simulink model "ammclib_gflib_limit_s32k11x"  (Simulink 9.0)
settings: Solver=FixedStepDiscrete  StartTime=0.0  StopTime=5  FixedStep=0.1  RelTol=1e-3  EnableMultiTasking=on
InitFcn:
  | mbd_s32k_consistency_checks(bdroot(gcs));
undefined symbols (not defined in the file): LQFP, thumb
libraries: simulink x11, ammclib_bam_s32k11x x10, mbd_s32k1xx_ec_toolbox x2
Description:
  | This model tests the AMMCLIB GFLIB LIMIT blocks
  | 
  | Validation:
  | - Run the model in Simulation and check the results
  | - Open Freemaster (ammclib_gflib_limit_s32k11x.pmp) and compare the HW results against the Simulated ones
CloseFcn:
  | clear all;
settings Model: Creator=NXP MBDT Team  LastModifiedBy=nxf35172
settings DataIOCC: ExternalInput=off  InitialState=off  LimitDataPoints=on  SaveOutput=off  SignalLogging=off  SaveTime=off
settings OptimizationCC: DefaultParameterBehavior=Inlined  PassReuseOutputArgsAs=Individual arguments  LifeSpan=auto
settings DebuggingCC: SolverPrmCheckMsg=warning  InheritedTsInSrcMsg=none  SingleTaskRateTransMsg=error  IntegerOverflowMsg=none  ParameterPrecisionLossMsg=none  ParameterTunabilityLossMsg=error  UnconnectedInputMsg=error  UnconnectedOutputMsg=error  UnconnectedLineMsg=error  AllowSymbolicDim=off  UnknownTsInhSupMsg=error  StateNameClashWarn=warning
settings HardwareCC: ProdLargestAtomicInteger=Long  ProdLargestAtomicFloat=Double  ProdIntDivRoundTo=Zero  ProdEndianess=LittleEndian  ProdHWDeviceType=ARM Compatible->ARM Cortex
settings SFSimCC: MATLABDynamicMemAlloc=off
settings RTWCC: SystemTargetFile=mbd_s32k.tlc  MakeCommand=mbd_s32k_make_rtw COPY_MDLREF_INCLUDES=0  TemplateMakefile=mbd_s32k.tmf  Description=Model Based Design Toolbox S32K14x Code Generation Target  GenerateReport=on  IncludeHyperlinkInReport=on  LaunchReport=on  GenerateTraceInfo=on  GenerateTraceReport=on  GenerateTraceReportSl=on  GenerateTraceReportSf=on  GenerateTraceReportEml=on
settings CodeAppCC: ForceParamTrailComments=on  IgnoreCustomStorageClasses=off  OperatorAnnotations=on  SimulinkDataObjDesc=on  SFDataObjDesc=on  InsertBlockDesc=on  StateflowObjectComments=off
settings STFCustomTargetCC: MultiwordLength=256  ModelReferenceCompliant=off  CombineOutputUpdateFcns=on  ERTCustomFileBanners=on  SupportContinuousTime=off  SupportNonInlinedSFcns=off  RemoveResetFunc=on  MATLABClassNameForMDSCustomization=Simulink.SoftwareTarget.ERTCustomization  GRTInterface=off  SystemTargetFile=mbd_s32k.tlc
settings ERTTargetCC: ModelReferenceCompliant=off  ParMdlRefBuildCompliant=off  CompOptLevelCompliant=off  ConcurrentExecutionCompliant=off  ModelStepFunctionPrototypeControlCompliant=off  CPPClassGenCompliant=off  UseToolchainInfoCompliant=off  InlinedParameterPlacement=NonHierarchical  ERTCustomFileTemplate=example_file_process.tlc

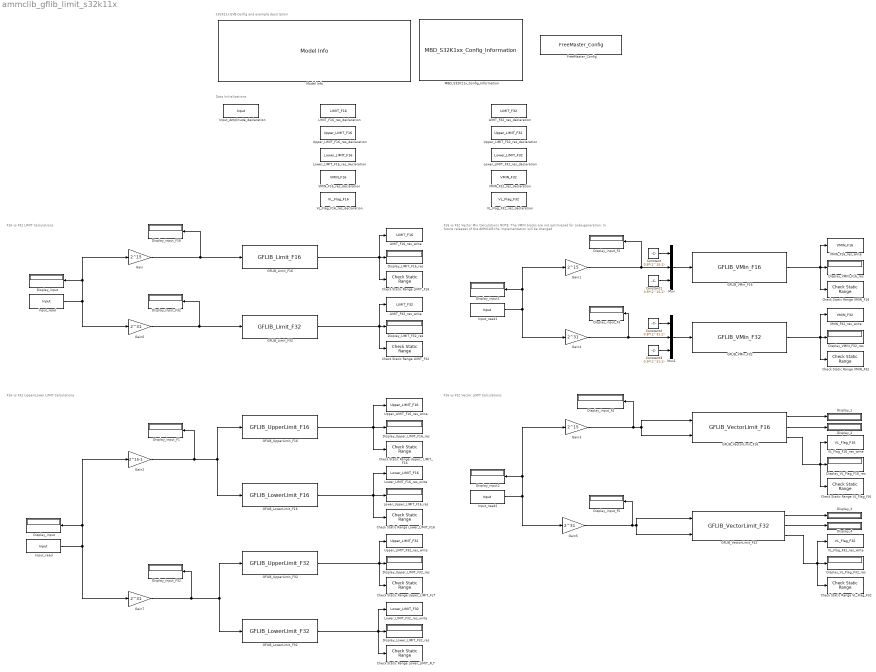
== system ammclib_gflib_limit_s32k11x ==
  note: S32K11x EVB Config and example description
  note: Data Initializations
  note: F16 vs F32 LIMIT Calculations
  note: F16 vs F32 Upper/Lower LIMIT Calculations
  note: F16 vs F32 Vector Min Calculations
      | NOTE: The VMIN blocks are not optimiezed for code-generation. In future releases of the AMMCLIB the implementation will be changed
  note: F16 vs F32 Vector LIMIT Calculations
  "Check Static Range LIMIT_F16 " : simulink/Model Verification/Check  Static Range  Description=-0.5*(2^15-1)-1 <= u <= 0.5*(2^15-1)+1  max=0.5*(2^15-1)+1  max_included=on  min=-0.5*(2^15-1)-1  min_included=on  enabled=on  stopWhenAssertionFail=on  export=off  icon=graphic
      settings: SourceProductName=Simulink  SourceProductBaseCode=SL
  Check Static Range LIMIT_F32 : simulink/Model Verification/Check  Static Range  Description=-0.5*(2^31-1)-1 <= u <= 0.5*(2^31-1)+1  max=0.5*(2^31-1)+1  max_included=on  min=-0.5*(2^31-1)-1  min_included=on  enabled=on  stopWhenAssertionFail=on  export=off  icon=graphic
      settings: SourceProductName=Simulink  SourceProductBaseCode=SL
  Check Static Range Lower_LIMIT_F16 : simulink/Model Verification/Check  Static Range  Description=-0.5*(2^15-1)-1 <= u <= (2^15-1)  max=(2^15-1)  max_included=on  min=-0.5*(2^15-1)-1  min_included=on  enabled=on  stopWhenAssertionFail=on  export=off  icon=graphic
      settings: SourceProductName=Simulink  SourceProductBaseCode=SL
  Check Static Range Lower_LIMIT_FLT : simulink/Model Verification/Check  Static Range  Description=-0.5*(2^31-1)-1 <= u <= (2^31-1)  max=(2^31-1)  max_included=on  min=-0.5*(2^31-1)-1  min_included=on  enabled=on  stopWhenAssertionFail=on  export=off  icon=graphic
      settings: SourceProductName=Simulink  SourceProductBaseCode=SL
  "Check Static Range Upper_ LIMIT_F16 " : simulink/Model Verification/Check  Static Range  Description=-(2^15-1) <= u <= 0.5*(2^15-1)+1  max=0.5*(2^15-1)+1  max_included=on  min=-(2^15-1)  min_included=on  enabled=on  stopWhenAssertionFail=on  export=off  icon=graphic
      settings: SourceProductName=Simulink  SourceProductBaseCode=SL
  Check Static Range Upper_LIMIT_FLT : simulink/Model Verification/Check  Static Range  Description=-(2^31-1) <= u <= 0.5*(2^31-1)+1  max=0.5*(2^31-1)+1  max_included=on  min=-(2^31-1)  min_included=on  enabled=on  stopWhenAssertionFail=on  export=off  icon=graphic
      settings: SourceProductName=Simulink  SourceProductBaseCode=SL
  Check Static Range VL_Flag_F32 : simulink/Model Verification/Check  Static Range  Description=0 <= u <= 1  max=1  max_included=on  min=0  min_included=on  enabled=on  stopWhenAssertionFail=on  export=off  icon=graphic
      settings: SourceProductName=Simulink  SourceProductBaseCode=SL
  Check Static Range VL_Flag_f16 : simulink/Model Verification/Check  Static Range  Description=0 <= u <= 1  max=1  max_included=on  min=0  min_included=on  enabled=on  stopWhenAssertionFail=on  export=off  icon=graphic
      settings: SourceProductName=Simulink  SourceProductBaseCode=SL
  Check Static Range VMIN_F16 : simulink/Model Verification/Check  Static Range  Description=0 <= u <= 2  max=2  max_included=on  min=0  min_included=on  enabled=on  stopWhenAssertionFail=on  export=off  icon=graphic
      settings: SourceProductName=Simulink  SourceProductBaseCode=SL
  Check Static Range VMIN_F32 : simulink/Model Verification/Check  Static Range  Description=0 <= u <= 2  max=2  max_included=on  min=0  min_included=on  enabled=on  stopWhenAssertionFail=on  export=off  icon=graphic
      settings: SourceProductName=Simulink  SourceProductBaseCode=SL
  Constant : Constant  Value=0.8*(2^15-1)  OutDataTypeStr=int16
  Constant1 : Constant  Value=0.9*(2^15-1)  OutDataTypeStr=int16
  Constant2 : Constant  Value=0.8*(2^31-1)  OutDataTypeStr=int32
  Constant3 : Constant  Value=0.9*(2^31-1)  OutDataTypeStr=int32
  Display_{1..4} (4 alike) : Display
  Display_LIMIT_F16_res : Display
  Display_LIMIT_F32_res : Display
  Display_Lower_LIMIT_F32_res : Display
  Display_Upper_LIMIT_F16_res : Display
  Display_Upper_LIMIT_F32_res : Display
  Display_VL_Flag_F16_res : Display
  Display_VL_Flag_F32_res : Display
  Display_VMIN_F16_res : Display
  Display_VMIN_F32_res : Display
  Display_input : Display
  "Display_input  " : Display
  Display_input1 : Display
  Display_input2 : Display
  Display_input_F{1..5,16,32} (7 alike) : Display
  "Display_input_F32  " : Display
  FreeMaster_Config : mbd_s32k1xx_ec_toolbox/Utility Blocks/FreeMaster_Config  interface=LPUART0  baudrate=19200  rxd=PTB0: [LPUART0_RX | Receive]  txd=PTB1: [LPUART0_TX | Transmit]  mode=Short Interrupt  isr_prio=1  show_adv_opts=on  use_scope=on  max_scope_vars=8  use_recorder=on  max_rec_vars=8  rec_buff_size=1024  rec_timebase=0 seconds  comm_buffer_size_auto=on  comm_buffer_size=255  comm_rqueue_size_default=on  comm_rqueue_size=32
  GFLIB_Limit_F16 : ammclib_bam_s32k11x/GFLIB/bam_f16/GFLIB_Limit_F16  f16UpperLimit=0.5*(2^15-1)  f16LowerLim=-0.5*(2^15-1)
  GFLIB_Limit_F32 : ammclib_bam_s32k11x/GFLIB/bam_f32/GFLIB_Limit_F32  f32UpperLimit=0.5*(2^31-1)  f32LowerLim=-0.5*(2^31-1)
  GFLIB_LowerLimit_F16 : ammclib_bam_s32k11x/GFLIB/bam_f16/GFLIB_LowerLimit_F16  f16LowerLim=-0.5*(2^15-1)
  GFLIB_LowerLimit_F32 : ammclib_bam_s32k11x/GFLIB/bam_f32/GFLIB_LowerLimit_F32  f32LowerLim=-0.5*(2^31-1)
  GFLIB_UpperLimit_F16 : ammclib_bam_s32k11x/GFLIB/bam_f16/GFLIB_UpperLimit_F16  f16UpperLim=0.5*(2^15-1)
  GFLIB_UpperLimit_F32 : ammclib_bam_s32k11x/GFLIB/bam_f32/GFLIB_UpperLimit_F32  f32UpperLim=0.5*(2^31-1)
  GFLIB_VMin_F16 : ammclib_bam_s32k11x/GFLIB/bam_f16/GFLIB_VMin_F16  N=3
  GFLIB_VMin_F32 : ammclib_bam_s32k11x/GFLIB/bam_f32/GFLIB_VMin_F32  N=3
  GFLIB_VectorLimit_F16 : ammclib_bam_s32k11x/GFLIB/bam_f16/GFLIB_VectorLimit_F16  f16Limit=0.5*(2^15-1)
  GFLIB_VectorLimit_F32 : ammclib_bam_s32k11x/GFLIB/bam_f32/GFLIB_VectorLimit_F32  f32Limit=0.5*(2^31-1)
  Gain : Gain  Gain=2^15  ParamDataTypeStr=int32  OutDataTypeStr=int16
  Gain1 : Gain  Gain=2^15  ParamDataTypeStr=int32  OutDataTypeStr=int16
  Gain2 : Gain  Gain=2^15-1  ParamDataTypeStr=int32  OutDataTypeStr=int16
  Gain3 : Gain  Gain=2^15  ParamDataTypeStr=int32  OutDataTypeStr=int16
  Gain{4..7} (4 alike) : Gain  Gain=2^31  ParamDataTypeStr=int32  OutDataTypeStr=int32
  Input_Amplitude_declaration : DataStoreMemory  Priority=1  DataStoreName=Input  WriteAfterWriteMsg=warning  WriteAfterReadMsg=warning  InitialValue=0.75  ShowAdditionalParam=off  OutMin=-1  OutMax=1  OutDataTypeStr=single
  Input_read : DataStoreRead  DataStoreName=Input
  "Input_read  " : DataStoreRead  DataStoreName=Input
  Input_read1 : DataStoreRead  DataStoreName=Input
  Input_read2 : DataStoreRead  DataStoreName=Input
  LIMIT_F16_res_declaration : DataStoreMemory  Priority=2  DataStoreName=LIMIT_F16  ReadBeforeWriteMsg=warning  WriteAfterWriteMsg=warning  WriteAfterReadMsg=warning  ShowAdditionalParam=off  OutDataTypeStr=int16
  LIMIT_F16_res_write : DataStoreWrite  DataStoreName=LIMIT_F16
  LIMIT_F32_res_declaration : DataStoreMemory  Priority=2  DataStoreName=LIMIT_F32  ReadBeforeWriteMsg=warning  WriteAfterWriteMsg=warning  WriteAfterReadMsg=warning  ShowAdditionalParam=off  OutDataTypeStr=int32
  LIMIT_F32_res_write : DataStoreWrite  DataStoreName=LIMIT_F32
  Lower_LIMIT_F16_res_declaration : DataStoreMemory  Priority=2  DataStoreName=Lower_LIMIT_F16  ReadBeforeWriteMsg=warning  WriteAfterWriteMsg=warning  WriteAfterReadMsg=warning  ShowAdditionalParam=off  OutDataTypeStr=int16
  Lower_LIMIT_F16_res_write : DataStoreWrite  DataStoreName=Lower_LIMIT_F16
  Lower_LIMIT_F32_res_declaration : DataStoreMemory  Priority=2  DataStoreName=Lower_LIMIT_F32  ReadBeforeWriteMsg=warning  WriteAfterWriteMsg=warning  WriteAfterReadMsg=warning  ShowAdditionalParam=off  OutDataTypeStr=int32
  Lower_LIMIT_F32_res_write : DataStoreWrite  DataStoreName=Lower_LIMIT_F32
  Lower_Upper_LIMIT_F16_res : Display
  MBD_S32K11x_Config_Information : mbd_s32k1xx_ec_toolbox/MBD_S32K1xx_Config_Information  mbdt_ver=0  disp_str=|  config_params=[]  mcu_target_name=S32K118  mcu_target_package=48-LQFP  mcu_target_sram_size=25KB  mcu_system_clock_freq=40  mcu_xtal_freq=External 40  mcu_steptick_timer=LPIT Channel 0  mcu_steptick_prio=3  ds_import_enable=on  target_compiler=GCC  target_memory=FLASH  gcc_target_compile_opts=-mcpu=cortex-m0plus -mthumb -O1 -g -gstrict-dwarf  gcc_target_assemble_opts=-mcpu=cortex-m0plus -mthumb -g  gcc_target_link_opts=-mcpu=cortex-m0plus -mthumb  gcc_target_default_lcf=on  gcc_target_user_lcf=S32K118_25_flash.ld  ghs_target_compile_opts=-mcpu=cortexm0plus -mthumb -fsoft -Ogeneral -Wundef -Wimplicit-int -Wshadow -Wtrigraphs --no_commons --gnu_asm -gnu99 -gdwarf-2 -G  ghs_target_assemble_opts=-mcpu=cortexm0plus -mthumb -fsoft --gnu_asm  ghs_target_link_opts=-mcpu=cortexm0plus -mthumb -fsoft  ghs_target_default_lcf=on  ghs_target_user_lcf=S32K118_25_flash.ld  iar_target_compile_opts=--thumb -Ol -e --debug --dlib_config normal  iar_target_assemble_opts=--thumb  iar_target_link_opts=--no_exceptions --vfe --inline  iar_target_default_lcf=on  iar_target_user_lcf=S32K118_25_flash.icf  pil_download_enable=off  rbl_download_enable=on  rbl_start_delay=5000  rbl_download_interface=OpenSDA  rbl_restart_request=off  rbl_com_port=Custom  rbl_com_port_custom=COM1  pil_download_rate=57600  pil_opensda_drive=Custom  pil_opensda_drive_custom=D  pil_uart_instance=0  pil_uart_rx=PTB0: [LPUART0_RX | Receive]  pil_uart_tx=PTB1: [LPUART0_TX | Transmit]  FTM_PWM_PcrCheckEnDis=on  FTM_Input_Edge_Inputs_PcrCheckEnDis=on  FTM_Dual_Edge_Inputs_PcrCheckEnDis=on  FTM_Quadrature_Inputs_PcrCheckEnDis=on  FTM_Hall_Sensor_Inputs_PcrCheckEnDis=on  LPTMR_PcrCheckEnDis=on  PIT_PcrCheckEnDis=on  RTC_PcrCheckEnDis=on  FlexCAN_PcrCheckEnDis=on  LIN_PcrCheckEnDis=on  FlexIO_PcrCheckEnDis=on  LPI2C_PcrCheckEnDis=on  LPSPI_PcrCheckEnDis=on  LPUART_PcrCheckEnDis=on  CMP_PcrCheckEnDis=on  GPIO_OutputPcrCheckEnDis=on  GPIO_InputPcrCheckEnDis=on  SBC_PcrCheckEnDis=on  AMMCLIB_PcrCheckEnDis=on  FM_PcrCheckEnDis=on  Profile_PcrCheckEnDis=on  ConfigParams_PcrCheckEnDis=on  ModelRef_PcrCheckEnDis=on  PDB0_PcrCheckEnDis=on  CSEc_PcrCheckEnDis=on  eDMA_PcrCheckEnDis=on  ADC_PcrCheckEnDis=on  WDOG_PcrCheckEnDis=on
      | Target : S32K144-64KB_SRAM
      | Package : 100-pin
      | System clock : 80 MHz
      | XTAL clock : External 8 MHz
      | Compiler : IAR
      | Target Type : FLASH
      | Download Code after build : off
      | Step Tick Interrupt Priority : 15
  Model Info : simulink/Model-Wide Utilities/Model Info  Frame=off  DisplayStringWithTags=|  HorizontalTextAlignment=Left  LeftAlignmentValue=0.02
      | Model Name: %<ModelName>
      | 
      | Description: %<Description>
  Mux : Mux  Inputs=3
  Mux1 : Mux  Inputs=3
  Upper_LIMIT_F16_res_declaration : DataStoreMemory  Priority=2  DataStoreName=Upper_LIMIT_F16  ReadBeforeWriteMsg=warning  WriteAfterWriteMsg=warning  WriteAfterReadMsg=warning  ShowAdditionalParam=off  OutDataTypeStr=int16
  Upper_LIMIT_F16_res_write : DataStoreWrite  DataStoreName=Upper_LIMIT_F16
  Upper_LIMIT_F32_res_declaration : DataStoreMemory  Priority=2  DataStoreName=Upper_LIMIT_F32  ReadBeforeWriteMsg=warning  WriteAfterWriteMsg=warning  WriteAfterReadMsg=warning  ShowAdditionalParam=off  OutDataTypeStr=int32
  Upper_LIMIT_F32_res_write : DataStoreWrite  DataStoreName=Upper_LIMIT_F32
  VL_Flag_F16_res_declaration : DataStoreMemory  Priority=2  DataStoreName=VL_Flag_F16  ReadBeforeWriteMsg=warning  WriteAfterWriteMsg=warning  WriteAfterReadMsg=warning  ShowAdditionalParam=off  OutDataTypeStr=boolean
  VL_Flag_F16_res_write : DataStoreWrite  DataStoreName=VL_Flag_F16
  VL_Flag_F32_res_declaration : DataStoreMemory  Priority=2  DataStoreName=VL_Flag_F32  ReadBeforeWriteMsg=warning  WriteAfterWriteMsg=warning  WriteAfterReadMsg=warning  ShowAdditionalParam=off  OutDataTypeStr=boolean
  VL_Flag_F32_res_write : DataStoreWrite  DataStoreName=VL_Flag_F32
  VMIN_F16_res_declaration : DataStoreMemory  Priority=2  DataStoreName=VMIN_F16  ReadBeforeWriteMsg=warning  WriteAfterWriteMsg=warning  WriteAfterReadMsg=warning  ShowAdditionalParam=off  OutDataTypeStr=uint16
  VMIN_F16_res_write : DataStoreWrite  DataStoreName=VMIN_F16
  VMIN_F32_res_declaration : DataStoreMemory  Priority=2  DataStoreName=VMIN_F32  ReadBeforeWriteMsg=warning  WriteAfterWriteMsg=warning  WriteAfterReadMsg=warning  ShowAdditionalParam=off  OutDataTypeStr=uint32
  VMIN_F32_res_write : DataStoreWrite  DataStoreName=VMIN_F32
  wires:
  Input_read/1 -> Gain6/1, Gain/1, Display_input/1
  Gain/1 -> Display_input_F16/1, GFLIB_Limit_F16/1
  GFLIB_Limit_F16/1 -> LIMIT_F16_res_write/1, Display_LIMIT_F16_res/1, "Check Static Range LIMIT_F16 "/1
  Gain6/1 -> GFLIB_Limit_F32/1, Display_input_F32/1
  GFLIB_Limit_F32/1 -> Check Static Range LIMIT_F32/1, LIMIT_F32_res_write/1, Display_LIMIT_F32_res/1
  "Input_read  "/1 -> Gain7/1, Gain2/1, "Display_input  "/1
  Gain2/1 -> GFLIB_LowerLimit_F16/1, GFLIB_UpperLimit_F16/1, Display_input_F1/1
  GFLIB_UpperLimit_F16/1 -> Upper_LIMIT_F16_res_write/1, Display_Upper_LIMIT_F16_res/1, "Check Static Range Upper_ LIMIT_F16 "/1
  Gain7/1 -> GFLIB_UpperLimit_F32/1, GFLIB_LowerLimit_F32/1, "Display_input_F32  "/1
  GFLIB_UpperLimit_F32/1 -> Check Static Range Upper_LIMIT_FLT/1, Upper_LIMIT_F32_res_write/1, Display_Upper_LIMIT_F32_res/1
  GFLIB_LowerLimit_F16/1 -> Check Static Range Lower_LIMIT_F16/1, Lower_LIMIT_F16_res_write/1, Lower_Upper_LIMIT_F16_res/1
  GFLIB_LowerLimit_F32/1 -> Check Static Range Lower_LIMIT_FLT/1, Lower_LIMIT_F32_res_write/1, Display_Lower_LIMIT_F32_res/1
  Gain1/1 -> Mux/2, Display_input_F2/1
  GFLIB_VMin_F16/1 -> Check Static Range VMIN_F16/1, VMIN_F16_res_write/1, Display_VMIN_F16_res/1
  GFLIB_VMin_F32/1 -> Check Static Range VMIN_F32/1, VMIN_F32_res_write/1, Display_VMIN_F32_res/1
  Mux/1 -> GFLIB_VMin_F16/1
  Constant/1 -> Mux/1
  Constant1/1 -> Mux/3
  Gain4/1 -> Mux1/2, Display_input_F3/1
  Mux1/1 -> GFLIB_VMin_F32/1
  Constant2/1 -> Mux1/1
  Constant3/1 -> Mux1/3
  Input_read2/1 -> Gain5/1, Gain3/1, Display_input2/1
  Gain3/1 -> GFLIB_VectorLimit_F16/1, GFLIB_VectorLimit_F16/2, Display_input_F4/1
  Gain5/1 -> GFLIB_VectorLimit_F32/1, GFLIB_VectorLimit_F32/2, Display_input_F5/1
  GFLIB_VectorLimit_F16/1 -> Display_1/1
  GFLIB_VectorLimit_F16/2 -> Display_2/1
  GFLIB_VectorLimit_F16/3 -> Check Static Range VL_Flag_f16/1, VL_Flag_F16_res_write/1, Display_VL_Flag_F16_res/1
  GFLIB_VectorLimit_F32/1 -> Display_3/1
  GFLIB_VectorLimit_F32/2 -> Display_4/1
  GFLIB_VectorLimit_F32/3 -> Check Static Range VL_Flag_F32/1, Display_VL_Flag_F32_res/1, VL_Flag_F32_res_write/1
  Input_read1/1 -> Gain4/1, Gain1/1, Display_input1/1
